simulink library "csu_imh_imu_hardware_lib"  (R2014b)
settings: Solver=ode45  SolverMode=SingleTasking  StartTime=0.0  StopTime=10.0  RelTol=1e-3
values from neighbouring files (symbols this model uses):
  imh_accel_range = 2*9.81    (= 19.62)    [csu_imh_imu_hardware_init.m]
  imh_accel_SF = 300/1e6    (= 0.0003)    [csu_imh_imu_hardware_init.m]
  imh_correlation_time = 100    [csu_imh_imu_hardware_init.m]
  imh_dt = sim_time_step_size    [csu_imh_imu_hardware_init.m]
  imh_gyro_g_sensitive = 2.471e-08 * [1 1 1]'    [csu_imh_imu_hardware_init.m]
  imh_gyro_range = 250*pi/180    (= 4.36332312999)    [csu_imh_imu_hardware_init.m]
  imh_gyro_SF = 100/1e6    (= 0.0001)    [csu_imh_imu_hardware_init.m]
  imh_gyro_vibe_sensitive = 5.04e-09 * [1 1 1]'    [csu_imh_imu_hardware_init.m]
libraries: util_common_lib x7, util_info_lib x1
settings Model: Creator=hcannon  LastModifiedBy=mstewart

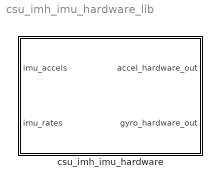
== system csu_imh_imu_hardware_lib ==
  csu_imh_imu_hardware : Subsystem

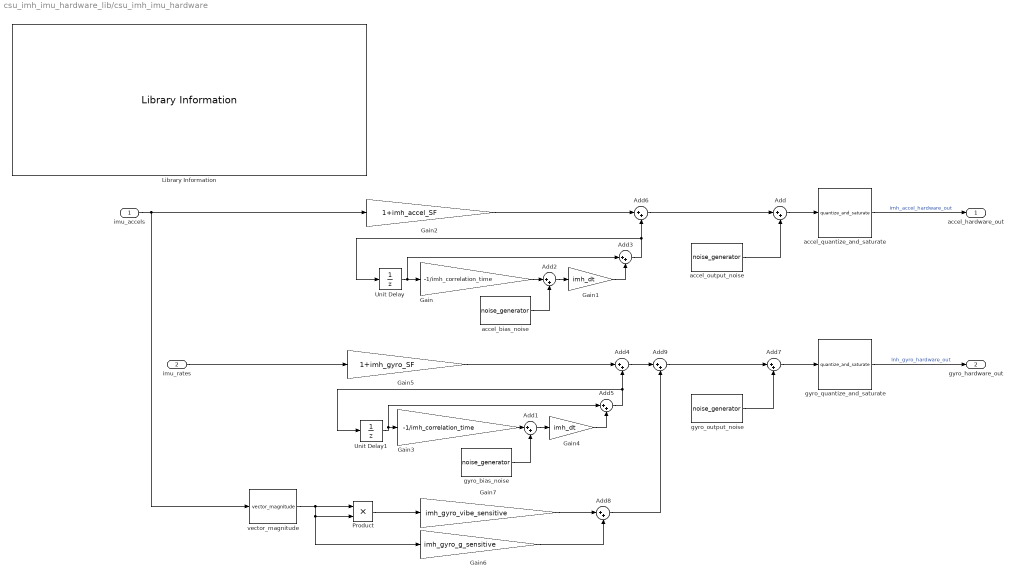
== system csu_imh_imu_hardware_lib/csu_imh_imu_hardware ==
  imu_accels : Inport
  imu_rates : Inport  Port=2
  Add{,1..9} (10 alike) : Sum  Inputs=|++
  Gain : Gain  Gain=-1/imh_correlation_time
  Gain1 : Gain  Gain=imh_dt
  Gain2 : Gain  Gain=1+imh_accel_SF
  Gain3 : Gain  Gain=-1/imh_correlation_time
  Gain4 : Gain  Gain=imh_dt
  Gain5 : Gain  Gain=1+imh_gyro_SF
  Gain6 : Gain  Gain=imh_gyro_g_sensitive
  Gain7 : Gain  Gain=imh_gyro_vibe_sensitive
  Library Information : util_info_lib/Library Information  owner='NONE'
  Product : Product  RndMeth=Zero
  Unit Delay : UnitDelay  SampleTime=-1
  Unit Delay1 : UnitDelay  SampleTime=-1
  accel_bias_noise : util_common_lib/noise_generator  std_dev=imh_accel_bias_noise_v  bias=imh_accel_bias_bias_v  seed=imh_accel_bias_seed_v  on=imh_accel_noise_on  sample_time=sim_time_step_size
  accel_output_noise : util_common_lib/noise_generator  std_dev=imh_accel_noise_v  bias=imh_accel_bias_v  seed=imh_accel_seed_v  on=imh_accel_noise_on  sample_time=sim_time_step_size
  accel_quantize_and_saturate : util_common_lib/quantize_and_saturate  RES=imh_accel_sensitivity  OPER=truncate  out_min=-imh_accel_range  out_max=imh_accel_range
  gyro_bias_noise : util_common_lib/noise_generator  std_dev=imh_gyro_bias_noise_v  bias=imh_gyro_bias_bias_v  seed=imh_gyro_bias_seed_v  on=imh_gyro_noise_on  sample_time=sim_time_step_size
  gyro_output_noise : util_common_lib/noise_generator  std_dev=imh_gyro_noise_v  bias=imh_gyro_bias_v  seed=imh_gyro_seed_v  on=imh_gyro_noise_on  sample_time=sim_time_step_size
  gyro_quantize_and_saturate : util_common_lib/quantize_and_saturate  RES=imh_gyro_sensitivity  OPER=truncate  out_min=-imh_gyro_range  out_max=imh_gyro_range
  vector_magnitude : util_common_lib/vector_magnitude  SystemSampleTime=-1
  accel_hardware_out : Outport
  gyro_hardware_out : Outport  Port=2
  wires:
  Add8/1 -> Add9/2
  Add9/1 -> Add7/1
  Add4/1 -> Add9/1
  Gain6/1 -> Add8/2
  Gain7/1 -> Add8/1
  Product/1 -> Gain7/1
  vector_magnitude/1 -> Gain6/1, Product/2, Product/1
  Add6/1 -> Add/1
  Gain2/1 -> Add6/1
  Gain5/1 -> Add4/1
  Add/1 -> accel_quantize_and_saturate/1
  accel_quantize_and_saturate/1 -> accel_hardware_out/1  "imh_accel_hardware_out"
  gyro_quantize_and_saturate/1 -> gyro_hardware_out/1  "lnh_gyro_hardware_out"
  accel_output_noise/1 -> Add/2
  Add2/1 -> Gain1/1
  Gain1/1 -> Add3/2
  Unit Delay/1 -> Gain/1, Add3/1
  Add3/1 -> Add6/2, Unit Delay/1
  imu_accels/1 -> Gain2/1, vector_magnitude/1
  Gain/1 -> Add2/1
  accel_bias_noise/1 -> Add2/2
  Add1/1 -> Gain4/1
  Gain4/1 -> Add5/2
  Unit Delay1/1 -> Gain3/1, Add5/1
  Add5/1 -> Add4/2, Unit Delay1/1
  imu_rates/1 -> Gain5/1
  Gain3/1 -> Add1/1
  gyro_bias_noise/1 -> Add1/2
  Add7/1 -> gyro_quantize_and_saturate/1
  gyro_output_noise/1 -> Add7/2
